simulink model "test"  (R2012b)
settings: Solver=ode45  StartTime=0.0  StopTime=10.0  RelTol=1e-3
undefined symbols (not defined in the file or in its folder): cont
settings Model: Creator=admin  LastModifiedBy=admin

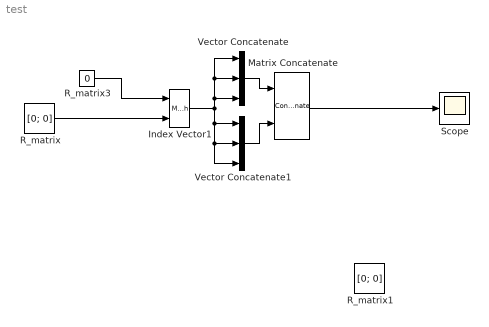
== system test ==
  Index Vector1 : MultiPortSwitch  DataPortOrder=Zero-based contiguous  Inputs=1  zeroidx=on
  Matrix Concatenate : Concatenate  Mode=Multidimensional array  ConcatenateDimension=2
  R_matrix : Constant  Value=[0; 0]  SampleTime=cont.LoopPeriod
  R_matrix1 : Constant  Value=[0; 0]  SampleTime=cont.LoopPeriod
  R_matrix3 : Constant  Value=0  SampleTime=cont.LoopPeriod
  Scope : Scope
  Vector Concatenate : Concatenate  NumInputs=3
  Vector Concatenate1 : Concatenate  NumInputs=3
  wires:
  R_matrix/1 -> Index Vector1/2
  R_matrix3/1 -> Index Vector1/1
  Matrix Concatenate/1 -> Scope/1
  Index Vector1/1 -> Vector Concatenate1/3, Vector Concatenate1/2, Vector Concatenate1/1, Vector Concatenate/3, Vector Concatenate/2, Vector Concatenate/1
  Vector Concatenate1/1 -> Matrix Concatenate/2
  Vector Concatenate/1 -> Matrix Concatenate/1
